simulink model "PROYECTO_III_SIMULINK_I"  (R2020b)
settings: Solver=VariableStepAuto  StartTime=0.0  StopTime=20  RelTol=1e-3
settings Model: Creator=NITRO  LastModifiedBy=NITRO

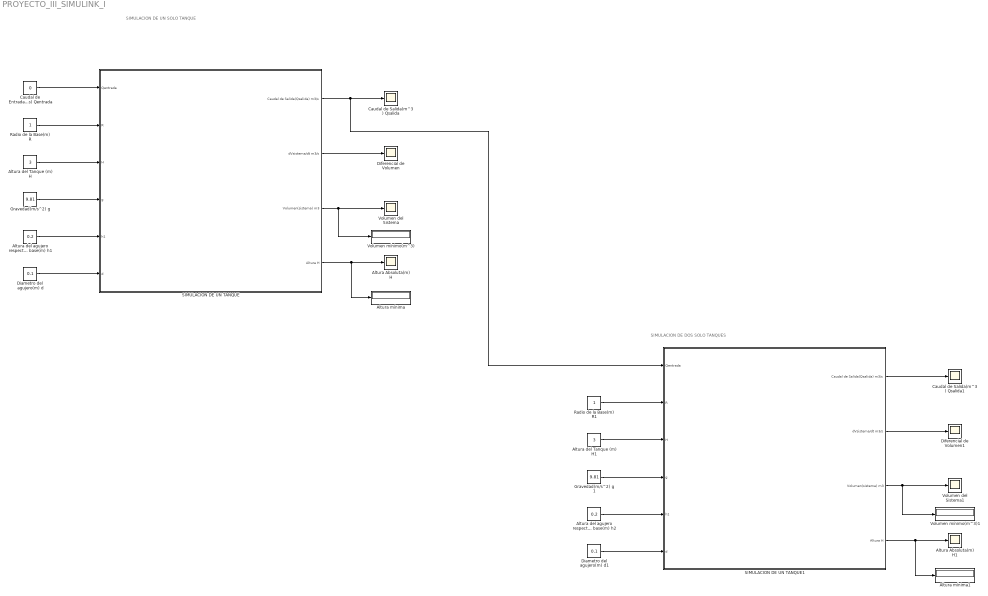
== system PROYECTO_III_SIMULINK_I ==
  note: SIMULACION DE UN SOLO TANQUE
  note: SIMULACION DE DOS SOLO TANQUES
  Altura Absoluta(m) H : Scope
  Altura Absoluta(m) H1 : Scope
  Altura del Tanque (m) H : Constant  Value=3
  Altura del Tanque (m) H1 : Constant  Value=3
  Altura del agujero respecto de la base(m) h1 : Constant  Value=0.2
  Altura del agujero respecto de la base(m) h2 : Constant  Value=0.2
  Altura mínima : Display
  Altura mínima1 : Display
  "Caudal de Entrada(m3/s) Qentrada " : Constant  Value=0
  Caudal de Salida(m^3) Qsalida : Scope
  Caudal de Salida(m^3) Qsalida1 : Scope
  Diametro del agujero(m) d : Constant  Value=0.1
  Diametro del agujero(m) d1 : Constant  Value=0.1
  Diferencial de Volumen : Scope
  Diferencial de Volumen1 : Scope
  "Gravedad(m/s^2) g " : Constant  Value=9.81
  Gravedad(m/s^2) g 1 : Constant  Value=9.81
  Radio de la Base(m) R : Constant
  Radio de la Base(m) R1 : Constant
  SIMULACION DE UN TANQUE : Subsystem
      mask Display: image('$imagefile'); % Use "Edit Image" on toolstrip to change.
  SIMULACION DE UN TANQUE1 : Subsystem
      mask Display: image('$imagefile'); % Use "Edit Image" on toolstrip to change.
  Volumen del Sistema : Scope
  Volumen del Sistema1 : Scope
  Volumen mínimo(m^3) : Display
  Volumen mínimo(m^3)1 : Display
  wires:
  SIMULACION DE UN TANQUE/4(Altura H) -> Altura Absoluta(m) H/1, Altura mínima/1
  SIMULACION DE UN TANQUE/3(Volumen(sistema) m3) -> Volumen del Sistema/1, Volumen mínimo(m^3)/1
  "Caudal de Entrada(m3/s) Qentrada "/1 -> SIMULACION DE UN TANQUE/1(Qentrada)
  Radio de la Base(m) R/1 -> SIMULACION DE UN TANQUE/2(R)
  Altura del Tanque (m) H/1 -> SIMULACION DE UN TANQUE/3(H)
  "Gravedad(m/s^2) g "/1 -> SIMULACION DE UN TANQUE/4(g)
  Altura del agujero respecto de la base(m) h1/1 -> SIMULACION DE UN TANQUE/5(h1)
  Diametro del agujero(m) d/1 -> SIMULACION DE UN TANQUE/6(d)
  SIMULACION DE UN TANQUE/2(dVsistema/dt m3/s) -> Diferencial de Volumen/1
  SIMULACION DE UN TANQUE1/2(dVsistema/dt m3/s) -> Diferencial de Volumen1/1
  SIMULACION DE UN TANQUE1/1(Caudal de Salida(Qsalida) m3/s) -> Caudal de Salida(m^3) Qsalida1/1
  Diametro del agujero(m) d1/1 -> SIMULACION DE UN TANQUE1/6(d)
  Altura del agujero respecto de la base(m) h2/1 -> SIMULACION DE UN TANQUE1/5(h1)
  Gravedad(m/s^2) g 1/1 -> SIMULACION DE UN TANQUE1/4(g)
  Altura del Tanque (m) H1/1 -> SIMULACION DE UN TANQUE1/3(H)
  Radio de la Base(m) R1/1 -> SIMULACION DE UN TANQUE1/2(R)
  SIMULACION DE UN TANQUE/1(Caudal de Salida(Qsalida) m3/s) -> SIMULACION DE UN TANQUE1/1(Qentrada), Caudal de Salida(m^3) Qsalida/1
  SIMULACION DE UN TANQUE1/3(Volumen(sistema) m3) -> Volumen mínimo(m^3)1/1, Volumen del Sistema1/1
  SIMULACION DE UN TANQUE1/4(Altura H) -> Altura mínima1/1, Altura Absoluta(m) H1/1

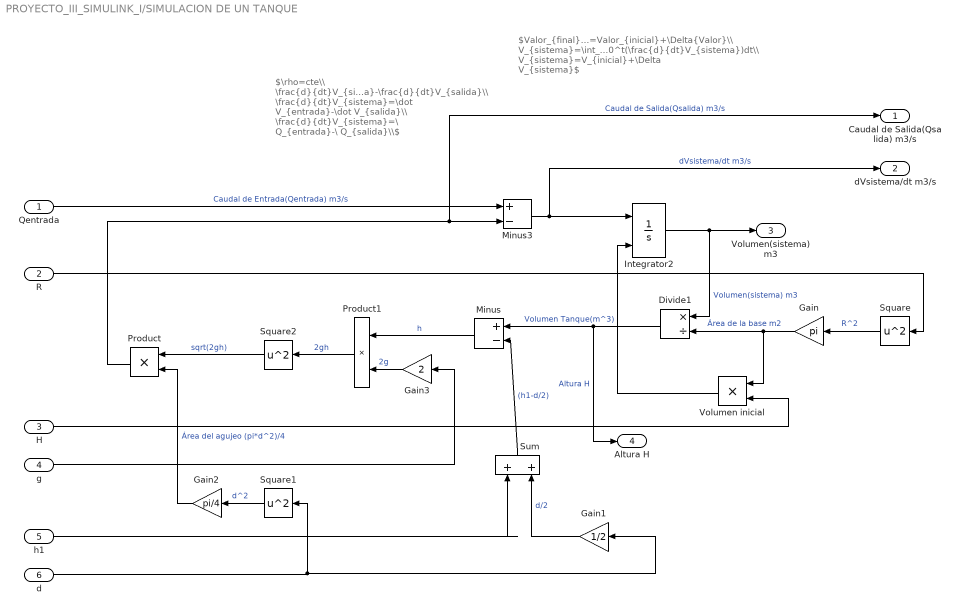
== system PROYECTO_III_SIMULINK_I/SIMULACION DE UN TANQUE ==
  note: $\rho=cte\\ \frac{d}{dt}V_{sistema}=\frac{d}{dt}V_{entrada}-\frac{d}{dt}V_{salida}\\ \frac{d}{dt}V_{sistema}=\dot V_{entrada}-\dot V_{salida}\\ \frac{d}{dt}V_{sistema}=\ Q_{entrada}-\ Q_{salida}\\$
  note: $Valor_{final}=Valor_{inicial}+\Delta{Valor}\\ V_{sistema}=\int_0^t(\frac{d}{dt}V_{sistema})dt\\ V_{sistema}=V_{inicial}+\Delta V_{sistema}$
  Qentrada : Inport
  R : Inport  Port=2
  H : Inport  Port=3
  g : Inport  Port=4
  h1 : Inport  Port=5
  d : Inport  Port=6
  Divide1 : Product  Inputs=*/
  Gain : Gain  Gain=pi
  Gain1 : Gain  Gain=1/2
  Gain2 : Gain  Gain=pi/4
  Gain3 : Gain  Gain=2
  Integrator2 : Integrator  InitialConditionSource=external
  Minus : Sum  Inputs=+-
  Minus3 : Sum  Inputs=+-
  Product : Product
  Product1 : Product
  Square : Math  Operator=square  SaturateOnIntegerOverflow=on
  Square1 : Math  Operator=square  SaturateOnIntegerOverflow=on
  Square2 : Math  Operator=square  SaturateOnIntegerOverflow=on
  Sum : Sum  Inputs=|++
  Volumen inicial : Product
  Caudal de Salida(Qsalida) m3/s : Outport
  dVsistema/dt m3/s : Outport  Port=2
  Volumen(sistema) m3 : Outport  Port=3
  Altura H : Outport  Port=4
  wires:
  Square1/1 -> Gain2/1  "d^2"
  Divide1/1 -> Altura H/1, Minus/1  "Altura H"
  Square/1 -> Gain/1  "R^2"
  Minus/1 -> Product1/1  "h"
  d/1 -> Square1/1, Gain1/1
  Gain1/1 -> Sum/2  "d/2"
  Volumen inicial/1 -> Integrator2/2  "Volumen Tanque(m^3)"
  Integrator2/1 -> Volumen(sistema) m3/1, Divide1/1  "Volumen(sistema) m3"
  Gain3/1 -> Product1/2  "2g"
  Gain/1 -> Volumen inicial/1, Divide1/2  "Área de la base m2"
  Product1/1 -> Square2/1  "2gh"
  h1/1 -> Sum/1
  Sum/1 -> Minus/2  "(h1-d/2)"
  g/1 -> Gain3/1
  Minus3/1 -> dVsistema/dt m3/s/1, Integrator2/1  "dVsistema/dt m3/s"
  Square2/1 -> Product/1  "sqrt(2gh)"
  R/1 -> Square/1
  Product/1 -> Caudal de Salida(Qsalida) m3/s/1, Minus3/2  "Caudal de Salida(Qsalida) m3/s"
  Gain2/1 -> Product/2  "Área del agujeo (pi*d^2)/4"
  Qentrada/1 -> Minus3/1  "Caudal de Entrada(Qentrada) m3/s"
  H/1 -> Volumen inicial/2

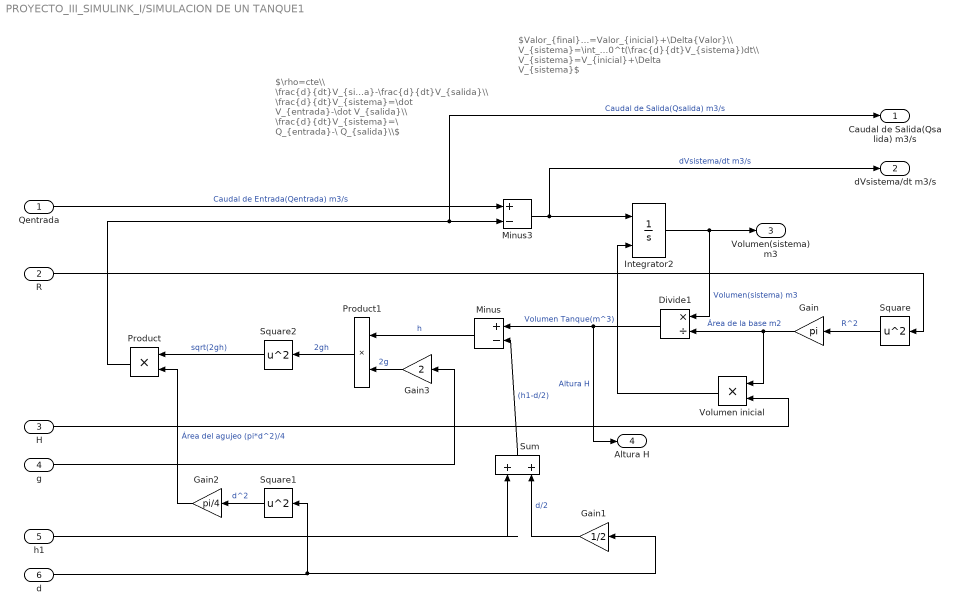
== system PROYECTO_III_SIMULINK_I/SIMULACION DE UN TANQUE1 ==
  note: $Valor_{final}=Valor_{inicial}+\Delta{Valor}\\ V_{sistema}=\int_0^t(\frac{d}{dt}V_{sistema})dt\\ V_{sistema}=V_{inicial}+\Delta V_{sistema}$
  note: $\rho=cte\\ \frac{d}{dt}V_{sistema}=\frac{d}{dt}V_{entrada}-\frac{d}{dt}V_{salida}\\ \frac{d}{dt}V_{sistema}=\dot V_{entrada}-\dot V_{salida}\\ \frac{d}{dt}V_{sistema}=\ Q_{entrada}-\ Q_{salida}\\$
  Qentrada : Inport
  R : Inport  Port=2
  H : Inport  Port=3
  g : Inport  Port=4
  h1 : Inport  Port=5
  d : Inport  Port=6
  Divide1 : Product  Inputs=*/
  Gain : Gain  Gain=pi
  Gain1 : Gain  Gain=1/2
  Gain2 : Gain  Gain=pi/4
  Gain3 : Gain  Gain=2
  Integrator2 : Integrator  InitialConditionSource=external
  Minus : Sum  Inputs=+-
  Minus3 : Sum  Inputs=+-
  Product : Product
  Product1 : Product
  Square : Math  Operator=square  SaturateOnIntegerOverflow=on
  Square1 : Math  Operator=square  SaturateOnIntegerOverflow=on
  Square2 : Math  Operator=square  SaturateOnIntegerOverflow=on
  Sum : Sum  Inputs=|++
  Volumen inicial : Product
  Caudal de Salida(Qsalida) m3/s : Outport
  dVsistema/dt m3/s : Outport  Port=2
  Volumen(sistema) m3 : Outport  Port=3
  Altura H : Outport  Port=4
  wires:
  H/1 -> Volumen inicial/2
  Qentrada/1 -> Minus3/1  "Caudal de Entrada(Qentrada) m3/s"
  Gain2/1 -> Product/2  "Área del agujeo (pi*d^2)/4"
  Product/1 -> Minus3/2, Caudal de Salida(Qsalida) m3/s/1  "Caudal de Salida(Qsalida) m3/s"
  R/1 -> Square/1
  Square2/1 -> Product/1  "sqrt(2gh)"
  Minus3/1 -> Integrator2/1, dVsistema/dt m3/s/1  "dVsistema/dt m3/s"
  g/1 -> Gain3/1
  Sum/1 -> Minus/2  "(h1-d/2)"
  h1/1 -> Sum/1
  Product1/1 -> Square2/1  "2gh"
  Gain/1 -> Divide1/2, Volumen inicial/1  "Área de la base m2"
  Gain3/1 -> Product1/2  "2g"
  Integrator2/1 -> Divide1/1, Volumen(sistema) m3/1  "Volumen(sistema) m3"
  Volumen inicial/1 -> Integrator2/2  "Volumen Tanque(m^3)"
  Gain1/1 -> Sum/2  "d/2"
  d/1 -> Gain1/1, Square1/1
  Minus/1 -> Product1/1  "h"
  Square/1 -> Gain/1  "R^2"
  Divide1/1 -> Minus/1, Altura H/1  "Altura H"
  Square1/1 -> Gain2/1  "d^2"
